simulink model "gravityLoad"  (R2018a)
settings: Solver=VariableStepAuto  StartTime=0.0  StopTime=10.0  RelTol=1e-3
settings Model: Creator=pei-T  LastModifiedBy=pei-T

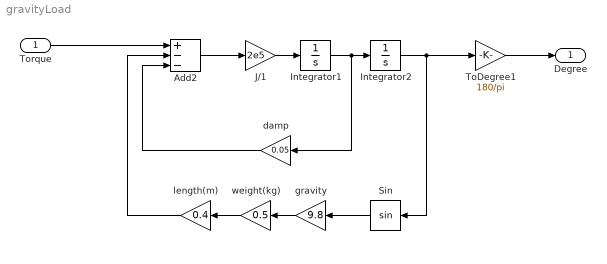
== system gravityLoad ==
  Torque : Inport
  Add2 : Sum  Inputs=+--
  Integrator1 : Integrator
  Integrator2 : Integrator
  J/1 : Gain  Gain=2e5
  Sin : Trigonometry
  ToDegree1 : Gain  Gain=180/pi
  damp : Gain  Gain=0.05
  gravity : Gain  Gain=9.8
  length(m) : Gain  Gain=0.4
  weight(kg) : Gain  Gain=0.5
  Degree : Outport
  wires:
  Sin/1 -> gravity/1
  Torque/1 -> Add2/1
  Add2/1 -> J/1/1
  Integrator2/1 -> Sin/1, ToDegree1/1
  gravity/1 -> weight(kg)/1
  weight(kg)/1 -> length(m)/1
  length(m)/1 -> Add2/2
  damp/1 -> Add2/3
  ToDegree1/1 -> Degree/1
  Integrator1/1 -> damp/1, Integrator2/1
  J/1/1 -> Integrator1/1
